simulink library "MSC_coder_lib"  (Simulink 8.6)
settings: Solver=ode45  StartTime=0.0  StopTime=10.0  RelTol=1e-3
undefined symbols (not defined in the file or in its folder): msc
libraries: dspmtrx3 x17, commsequence2 x12, commcnvcod2 x6, commblkintrlv2 x5, dspbuff3 x4, commdigbbndam3 x3, MSC_coder_lib x1
settings Model: Creator=Kevin  LastModifiedBy=dtdsv

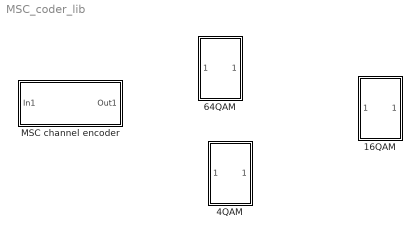
== system MSC_coder_lib ==
  16QAM : Subsystem
  4QAM : Subsystem
  64QAM : Subsystem
  MSC channel encoder : Subsystem  BlockChoice=16QAM
      settings: TemplateBlock=self  MemberBlocks=16QAM,4QAM,64QAM

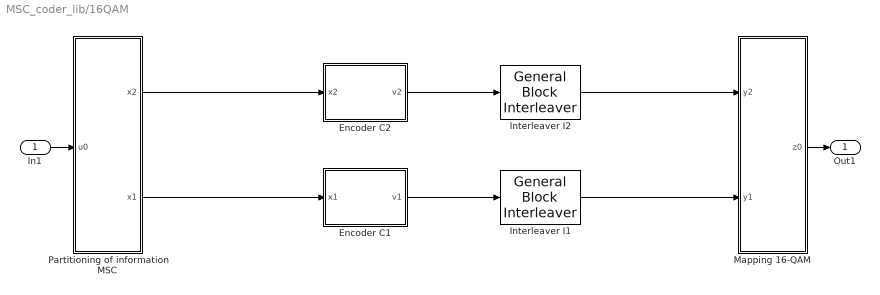
== system MSC_coder_lib/16QAM ==
  In1 : Inport
  Encoder C1 : Subsystem
  Encoder C2 : Subsystem
  Interleaver I1 : commblkintrlv2/General Block Interleaver  permutationVectorSource=Dialog  elements=msc.interleave_P0
  Interleaver I2 : commblkintrlv2/General Block Interleaver  permutationVectorSource=Dialog  elements=msc.interleave_P1
  Mapping 16-QAM : Subsystem
  Partitioning of information MSC : Subsystem
  Out1 : Outport
  wires:
  Encoder C2/1(v2) -> Interleaver I2/1
  Partitioning of information MSC/2(x1) -> Encoder C1/1(x1)
  Partitioning of information MSC/1(x2) -> Encoder C2/1(x2)
  Encoder C1/1(v1) -> Interleaver I1/1
  Interleaver I2/1 -> Mapping 16-QAM/1(y2)
  Interleaver I1/1 -> Mapping 16-QAM/2(y1)
  Mapping 16-QAM/1(z0) -> Out1/1
  In1/1 -> Partitioning of information MSC/1(u0)

== system MSC_coder_lib/4QAM ==
  In1 : Inport
  Demapping 4-QAM : commdigbbndam3/Rectangular QAM Modulator Baseband  M=MSC_QAM  InType=Bit  Enc=User-defined  Mapping=msc.qam_map  PowType=Min. distance between symbols  MinDist=msc.qam_norm  AvgPow=1  PeakPow=1  Ph=0  outDtype=double  outWordLen=16  outUDDataType=sfix(16)  outFracLenMode=Best precision  outFracLen=15
  Encoder C0 : Subsystem
  Interleaver I0 : commblkintrlv2/General Block Interleaver  permutationVectorSource=Dialog  elements=msc.interleave_P0
  Out1 : Outport
  wires:
  Encoder C0/1(v2) -> Interleaver I0/1
  Interleaver I0/1 -> Demapping 4-QAM/1
  Demapping 4-QAM/1 -> Out1/1
  In1/1 -> Encoder C0/1(x2)

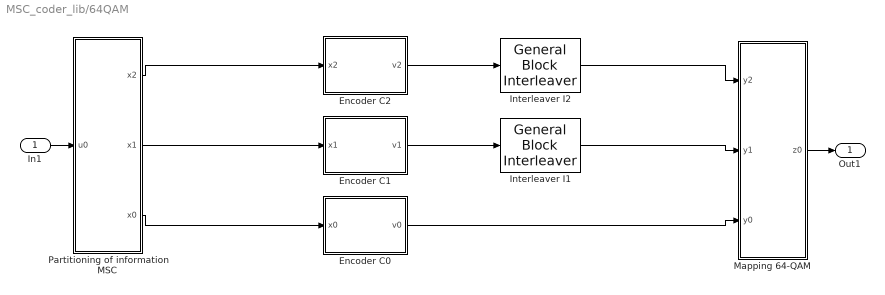
== system MSC_coder_lib/64QAM ==
  In1 : Inport
  Encoder C0 : Subsystem
  Encoder C1 : Subsystem
  Encoder C2 : Subsystem
  Interleaver I1 : commblkintrlv2/General Block Interleaver  permutationVectorSource=Dialog  elements=msc.interleave_P1
  Interleaver I2 : commblkintrlv2/General Block Interleaver  permutationVectorSource=Dialog  elements=msc.interleave_P2
  Mapping 64-QAM : Subsystem
  Partitioning of information MSC : Subsystem
  Out1 : Outport
  wires:
  Partitioning of information MSC/3(x0) -> Encoder C0/1(x0)
  Encoder C0/1(v0) -> Mapping 64-QAM/3(y0)
  Encoder C2/1(v2) -> Interleaver I2/1
  Partitioning of information MSC/2(x1) -> Encoder C1/1(x1)
  Partitioning of information MSC/1(x2) -> Encoder C2/1(x2)
  Encoder C1/1(v1) -> Interleaver I1/1
  Interleaver I2/1 -> Mapping 64-QAM/1(y2)
  Interleaver I1/1 -> Mapping 64-QAM/2(y1)
  In1/1 -> Partitioning of information MSC/1(u0)
  Mapping 64-QAM/1(z0) -> Out1/1

== system MSC_coder_lib/MSC channel encoder ==
  In1 : Inport
  16QAM : MSC_coder_lib/16QAM
  Out1 : Outport
  wires:
  In1/1 -> 16QAM/1
  16QAM/1 -> Out1/1

== system MSC_coder_lib/16QAM/Encoder C1 ==
  x1 : Inport
  "Conv. Encoder " : commcnvcod2/Convolutional Encoder  trellis=conv_poly  opMode=Terminate trellis by appending bits  hasIniStPort=off  hasFinStPort=off  usePuncVector=off  punctureVector=punc_rp35  reset=Unused parameter value
  Puncturing : Subsystem
  v1 : Outport
  wires:
  Puncturing/1(Out1) -> v1/1
  x1/1 -> "Conv. Encoder "/1
  "Conv. Encoder "/1 -> Puncturing/1(In1)

== system MSC_coder_lib/16QAM/Encoder C2 ==
  x2 : Inport
  Conv. Encoder : commcnvcod2/Convolutional Encoder  trellis=conv_poly  opMode=Terminate trellis by appending bits  DelayedResetAction=off  hasIniStPort=off  hasFinStPort=off  usePuncVector=off  punctureVector=punc_rp35  reset=Unused parameter value
  Puncturing : Subsystem
  v2 : Outport
  wires:
  Puncturing/1(Out1) -> v2/1
  x2/1 -> Conv. Encoder/1
  Conv. Encoder/1 -> Puncturing/1(In1)

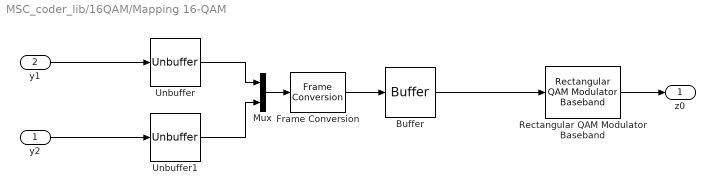
== system MSC_coder_lib/16QAM/Mapping 16-QAM ==
  y2 : Inport
  y1 : Inport  Port=2
  Buffer : Buffer  N=4*msc.NmbQAMcells
  Frame Conversion : FrameConversion  InheritSamplingMode=off
  Mux : Mux  Inputs=2
  Rectangular QAM Modulator Baseband : commdigbbndam3/Rectangular QAM Modulator Baseband  M=MSC_QAM  InType=Bit  Enc=User-defined  Mapping=msc.qam_map  PowType=Min. distance between symbols  MinDist=msc.qam_norm  AvgPow=1  PeakPow=1  Ph=0  outDtype=double  outWordLen=16  outUDDataType=sfix(16)  outFracLenMode=Best precision  outFracLen=15
  Unbuffer : Unbuffer
  Unbuffer1 : Unbuffer
  z0 : Outport
  wires:
  Rectangular QAM Modulator Baseband/1 -> z0/1
  Mux/1 -> Frame Conversion/1
  Unbuffer1/1 -> Mux/2
  Unbuffer/1 -> Mux/1
  Frame Conversion/1 -> Buffer/1
  Buffer/1 -> Rectangular QAM Modulator Baseband/1
  y1/1 -> Unbuffer/1
  y2/1 -> Unbuffer1/1

== system MSC_coder_lib/16QAM/Partitioning of information MSC ==
  u0 : Inport
  Submatrix3 : dspmtrx3/Submatrix  RowSpan=Range of rows  RowStartMode=Index  RowStartIndex=msc.ind_M1  RowEndMode=Last  RowEndIndex=msc.ind_M1  ColSpan=All columns  ColStartMode=First  ColStartIndex=1  ColEndMode=Last  ColEndIndex=1
  Submatrix4 : dspmtrx3/Submatrix  RowSpan=Range of rows  RowStartMode=First  RowStartIndex=msc.ind_M0  RowEndMode=Index  RowEndIndex=msc.ind_M0  ColSpan=All columns  ColStartMode=First  ColStartIndex=1  ColEndMode=Last  ColEndIndex=1
  x2 : Outport
  x1 : Outport  Port=2
  wires:
  Submatrix4/1 -> x1/1
  Submatrix3/1 -> x2/1
  u0/1 -> Submatrix3/1, Submatrix4/1

== system MSC_coder_lib/4QAM/Encoder C0 ==
  x2 : Inport
  Conv. Encoder : commcnvcod2/Convolutional Encoder  trellis=conv_poly  opMode=Terminate trellis by appending bits  hasIniStPort=off  hasFinStPort=off  usePuncVector=off  punctureVector=punc_rp35  reset=Unused parameter value
  Puncturing : Subsystem
  v2 : Outport
  wires:
  Puncturing/1(Out1) -> v2/1
  x2/1 -> Conv. Encoder/1
  Conv. Encoder/1 -> Puncturing/1(In1)

== system MSC_coder_lib/64QAM/Encoder C0 ==
  x0 : Inport
  Conv. Encoder : commcnvcod2/Convolutional Encoder  trellis=conv_poly  opMode=Terminate trellis by appending bits  hasIniStPort=off  hasFinStPort=off  usePuncVector=off  punctureVector=punc_rp35  reset=Unused parameter value
  Puncturing : Subsystem
  v0 : Outport
  wires:
  Conv. Encoder/1 -> Puncturing/1(In1)
  x0/1 -> Conv. Encoder/1
  Puncturing/1(Out1) -> v0/1

== system MSC_coder_lib/64QAM/Encoder C1 ==
  x1 : Inport
  "Conv. Encoder " : commcnvcod2/Convolutional Encoder  trellis=conv_poly  opMode=Terminate trellis by appending bits  hasIniStPort=off  hasFinStPort=off  usePuncVector=off  punctureVector=punc_rp35  reset=Unused parameter value
  Puncturing : Subsystem
  v1 : Outport
  wires:
  Puncturing/1(Out1) -> v1/1
  x1/1 -> "Conv. Encoder "/1
  "Conv. Encoder "/1 -> Puncturing/1(In1)

== system MSC_coder_lib/64QAM/Encoder C2 ==
  x2 : Inport
  Conv. Encoder : commcnvcod2/Convolutional Encoder  trellis=conv_poly  opMode=Terminate trellis by appending bits  hasIniStPort=off  hasFinStPort=off  usePuncVector=off  punctureVector=punc_rp35  reset=Unused parameter value
  Puncturing : Subsystem
  v2 : Outport
  wires:
  Puncturing/1(Out1) -> v2/1
  x2/1 -> Conv. Encoder/1
  Conv. Encoder/1 -> Puncturing/1(In1)

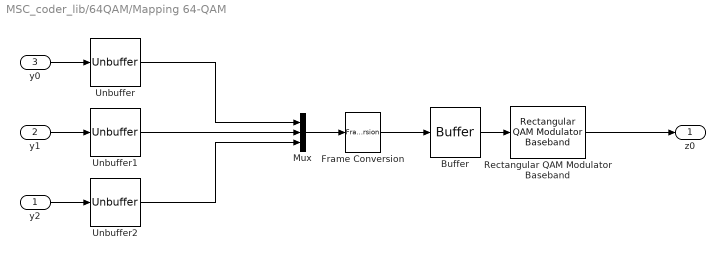
== system MSC_coder_lib/64QAM/Mapping 64-QAM ==
  y2 : Inport
  y1 : Inport  Port=2
  y0 : Inport  Port=3
  Buffer : dspbuff3/Buffer  N=6*msc.NmbQAMcells  V=0  ic=0
  Frame Conversion : FrameConversion  InheritSamplingMode=off
  Mux : Mux  Inputs=3
  Rectangular QAM Modulator Baseband : commdigbbndam3/Rectangular QAM Modulator Baseband  M=MSC_QAM  InType=Bit  Enc=User-defined  Mapping=msc.qam_map  PowType=Min. distance between symbols  MinDist=msc.qam_norm  AvgPow=1  PeakPow=1  Ph=0  outDtype=double  outWordLen=16  outUDDataType=sfix(16)  outFracLenMode=Best precision  outFracLen=15
  Unbuffer : dspbuff3/Unbuffer  ic=0
  Unbuffer1 : dspbuff3/Unbuffer  ic=0
  Unbuffer2 : dspbuff3/Unbuffer  ic=0
  z0 : Outport
  wires:
  Rectangular QAM Modulator Baseband/1 -> z0/1
  y0/1 -> Unbuffer/1
  y1/1 -> Unbuffer1/1
  y2/1 -> Unbuffer2/1
  Unbuffer/1 -> Mux/1
  Unbuffer1/1 -> Mux/2
  Unbuffer2/1 -> Mux/3
  Mux/1 -> Frame Conversion/1
  Buffer/1 -> Rectangular QAM Modulator Baseband/1
  Frame Conversion/1 -> Buffer/1

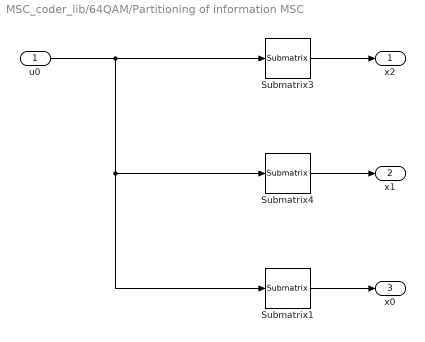
== system MSC_coder_lib/64QAM/Partitioning of information MSC ==
  u0 : Inport
  Submatrix1 : dspmtrx3/Submatrix  RowSpan=Range of rows  RowStartMode=First  RowStartIndex=msc.ind_M0  RowEndMode=Index  RowEndIndex=msc.ind_M0  ColSpan=All columns  ColStartMode=First  ColStartIndex=1  ColEndMode=Last  ColEndIndex=1
  Submatrix3 : dspmtrx3/Submatrix  RowSpan=Range of rows  RowStartMode=Offset from last  RowStartIndex=msc.ind_M2  RowEndMode=Last  RowEndIndex=msc.ind_M2  ColSpan=All columns  ColStartMode=First  ColStartIndex=1  ColEndMode=Last  ColEndIndex=1
  Submatrix4 : dspmtrx3/Submatrix  RowSpan=Range of rows  RowStartMode=Index  RowStartIndex=msc.ind_M0+1  RowEndMode=Index  RowEndIndex=msc.ind_M1  ColSpan=All columns  ColStartMode=First  ColStartIndex=1  ColEndMode=Last  ColEndIndex=1
  x2 : Outport
  x1 : Outport  Port=2
  x0 : Outport  Port=3
  wires:
  Submatrix1/1 -> x0/1
  Submatrix4/1 -> x1/1
  Submatrix3/1 -> x2/1
  u0/1 -> Submatrix1/1, Submatrix4/1, Submatrix3/1

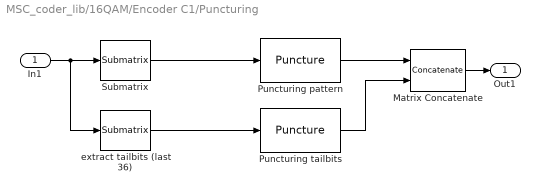
== system MSC_coder_lib/16QAM/Encoder C1/Puncturing ==
  In1 : Inport
  Matrix Concatenate : Concatenate  Mode=Multidimensional array
  Puncturing pattern : commsequence2/Puncture  punctureVector=msc.punc_pat0
  Puncturing tailbits : commsequence2/Puncture  punctureVector=msc.punc_tail0
  Submatrix : dspmtrx3/Submatrix  RowSpan=Range of rows  RowStartMode=First  RowStartIndex=1  RowEndMode=Offset from last  RowEndIndex=36  ColSpan=All columns  ColStartMode=First  ColStartIndex=1  ColEndMode=Last  ColEndIndex=1
  extract tailbits (last 36) : dspmtrx3/Submatrix  RowSpan=Range of rows  RowStartMode=Offset from last  RowStartIndex=35  RowEndMode=Last  RowEndIndex=35  ColSpan=All columns  ColStartMode=First  ColStartIndex=1  ColEndMode=Last  ColEndIndex=1
  Out1 : Outport
  wires:
  Matrix Concatenate/1 -> Out1/1
  Puncturing pattern/1 -> Matrix Concatenate/1
  Puncturing tailbits/1 -> Matrix Concatenate/2
  extract tailbits (last 36)/1 -> Puncturing tailbits/1
  Submatrix/1 -> Puncturing pattern/1
  In1/1 -> Submatrix/1, extract tailbits (last 36)/1

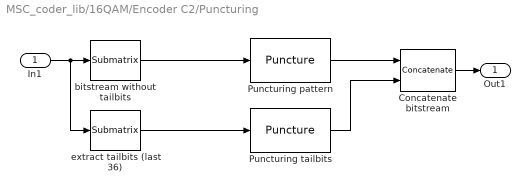
== system MSC_coder_lib/16QAM/Encoder C2/Puncturing ==
  In1 : Inport
  Concatenate bitstream : Concatenate  Mode=Multidimensional array
  Puncturing pattern : commsequence2/Puncture  punctureVector=msc.punc_pat1
  Puncturing tailbits : commsequence2/Puncture  punctureVector=msc.punc_tail1
  bitstream without tailbits : dspmtrx3/Submatrix  RowSpan=Range of rows  RowStartMode=First  RowStartIndex=1  RowEndMode=Offset from last  RowEndIndex=36  ColSpan=All columns  ColStartMode=First  ColStartIndex=1  ColEndMode=Last  ColEndIndex=1
  extract tailbits (last 36) : dspmtrx3/Submatrix  RowSpan=Range of rows  RowStartMode=Offset from last  RowStartIndex=35  RowEndMode=Last  RowEndIndex=35  ColSpan=All columns  ColStartMode=First  ColStartIndex=1  ColEndMode=Last  ColEndIndex=1
  Out1 : Outport
  wires:
  Concatenate bitstream/1 -> Out1/1
  In1/1 -> bitstream without tailbits/1, extract tailbits (last 36)/1
  Puncturing pattern/1 -> Concatenate bitstream/1
  Puncturing tailbits/1 -> Concatenate bitstream/2
  bitstream without tailbits/1 -> Puncturing pattern/1
  extract tailbits (last 36)/1 -> Puncturing tailbits/1

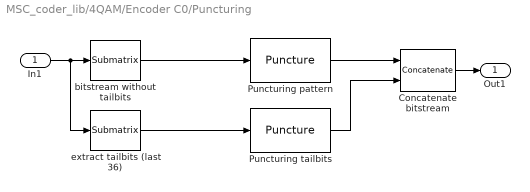
== system MSC_coder_lib/4QAM/Encoder C0/Puncturing ==
  In1 : Inport
  Concatenate bitstream : Concatenate  Mode=Multidimensional array
  Puncturing pattern : commsequence2/Puncture  punctureVector=msc.punc_pat0
  Puncturing tailbits : commsequence2/Puncture  punctureVector=msc.punc_tail0
  bitstream without tailbits : dspmtrx3/Submatrix  RowSpan=Range of rows  RowStartMode=First  RowStartIndex=1  RowEndMode=Offset from last  RowEndIndex=36  ColSpan=All columns  ColStartMode=First  ColStartIndex=1  ColEndMode=Last  ColEndIndex=1
  extract tailbits (last 36) : dspmtrx3/Submatrix  RowSpan=Range of rows  RowStartMode=Offset from last  RowStartIndex=35  RowEndMode=Last  RowEndIndex=35  ColSpan=All columns  ColStartMode=First  ColStartIndex=1  ColEndMode=Last  ColEndIndex=1
  Out1 : Outport
  wires:
  Concatenate bitstream/1 -> Out1/1
  In1/1 -> bitstream without tailbits/1, extract tailbits (last 36)/1
  Puncturing pattern/1 -> Concatenate bitstream/1
  Puncturing tailbits/1 -> Concatenate bitstream/2
  bitstream without tailbits/1 -> Puncturing pattern/1
  extract tailbits (last 36)/1 -> Puncturing tailbits/1

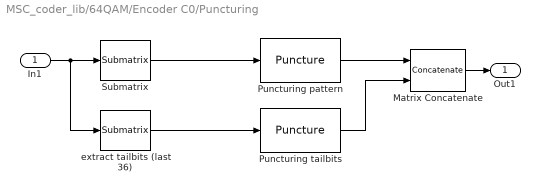
== system MSC_coder_lib/64QAM/Encoder C0/Puncturing ==
  In1 : Inport
  Matrix Concatenate : Concatenate  Mode=Multidimensional array
  Puncturing pattern : commsequence2/Puncture  punctureVector=msc.punc_pat0
  Puncturing tailbits : commsequence2/Puncture  punctureVector=msc.punc_tail0
  Submatrix : dspmtrx3/Submatrix  RowSpan=Range of rows  RowStartMode=First  RowStartIndex=1  RowEndMode=Offset from last  RowEndIndex=36  ColSpan=All columns  ColStartMode=First  ColStartIndex=1  ColEndMode=Last  ColEndIndex=1
  extract tailbits (last 36) : dspmtrx3/Submatrix  RowSpan=Range of rows  RowStartMode=Offset from last  RowStartIndex=35  RowEndMode=Last  RowEndIndex=35  ColSpan=All columns  ColStartMode=First  ColStartIndex=1  ColEndMode=Last  ColEndIndex=1
  Out1 : Outport
  wires:
  In1/1 -> extract tailbits (last 36)/1, Submatrix/1
  Submatrix/1 -> Puncturing pattern/1
  extract tailbits (last 36)/1 -> Puncturing tailbits/1
  Puncturing tailbits/1 -> Matrix Concatenate/2
  Puncturing pattern/1 -> Matrix Concatenate/1
  Matrix Concatenate/1 -> Out1/1

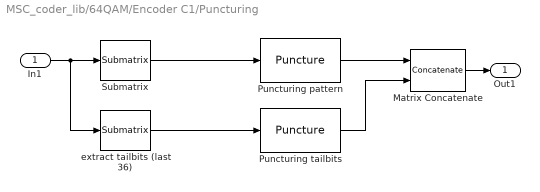
== system MSC_coder_lib/64QAM/Encoder C1/Puncturing ==
  In1 : Inport
  Matrix Concatenate : Concatenate  Mode=Multidimensional array
  Puncturing pattern : commsequence2/Puncture  punctureVector=msc.punc_pat1
  Puncturing tailbits : commsequence2/Puncture  punctureVector=msc.punc_tail1
  Submatrix : dspmtrx3/Submatrix  RowSpan=Range of rows  RowStartMode=First  RowStartIndex=1  RowEndMode=Offset from last  RowEndIndex=36  ColSpan=All columns  ColStartMode=First  ColStartIndex=1  ColEndMode=Last  ColEndIndex=1
  extract tailbits (last 36) : dspmtrx3/Submatrix  RowSpan=Range of rows  RowStartMode=Offset from last  RowStartIndex=35  RowEndMode=Last  RowEndIndex=35  ColSpan=All columns  ColStartMode=First  ColStartIndex=1  ColEndMode=Last  ColEndIndex=1
  Out1 : Outport
  wires:
  Matrix Concatenate/1 -> Out1/1
  Puncturing pattern/1 -> Matrix Concatenate/1
  Puncturing tailbits/1 -> Matrix Concatenate/2
  extract tailbits (last 36)/1 -> Puncturing tailbits/1
  Submatrix/1 -> Puncturing pattern/1
  In1/1 -> Submatrix/1, extract tailbits (last 36)/1

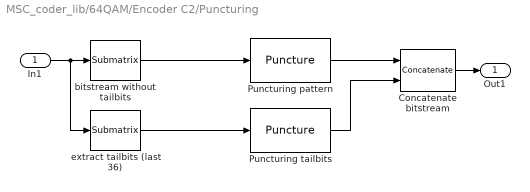
== system MSC_coder_lib/64QAM/Encoder C2/Puncturing ==
  In1 : Inport
  Concatenate bitstream : Concatenate  Mode=Multidimensional array
  Puncturing pattern : commsequence2/Puncture  punctureVector=msc.punc_pat2
  Puncturing tailbits : commsequence2/Puncture  punctureVector=msc.punc_tail2
  bitstream without tailbits : dspmtrx3/Submatrix  RowSpan=Range of rows  RowStartMode=First  RowStartIndex=1  RowEndMode=Offset from last  RowEndIndex=36  ColSpan=All columns  ColStartMode=First  ColStartIndex=1  ColEndMode=Last  ColEndIndex=1
  extract tailbits (last 36) : dspmtrx3/Submatrix  RowSpan=Range of rows  RowStartMode=Offset from last  RowStartIndex=35  RowEndMode=Last  RowEndIndex=35  ColSpan=All columns  ColStartMode=First  ColStartIndex=1  ColEndMode=Last  ColEndIndex=1
  Out1 : Outport
  wires:
  Concatenate bitstream/1 -> Out1/1
  In1/1 -> bitstream without tailbits/1, extract tailbits (last 36)/1
  Puncturing pattern/1 -> Concatenate bitstream/1
  Puncturing tailbits/1 -> Concatenate bitstream/2
  bitstream without tailbits/1 -> Puncturing pattern/1
  extract tailbits (last 36)/1 -> Puncturing tailbits/1
